simulink library "vmc"  (R2021b)
settings: Solver=VariableStepAuto  StartTime=0.0  StopTime=10.0  RelTol=1e-3
undefined symbols (not defined in the file or in its folder): AVMC_ACCDeltaTqIGain_X_kph, AVMC_ACCDeltaTqIGain_Y_mps2, AVMC_ACCDeltaTqPGain_X_kph, AVMC_ACCDeltaTqPGain_Y_kph, AVMC_ACCLongSteadyCtrl_X_kph, AVMC_AggressJerkPCT4AT_X_kph, AVMC_AggressJerkPCT_X_kph, AVMC_AggressLimitPCT4AT_X_kph, AVMC_AggressLimitPCT_X_kph, AVMC_CCLongSteadyCtrl_X_kph, AVMC_DISCDeltaTqIGain_X_kph, AVMC_DISCDeltaTqIGain_Y_mps2, AVMC_DISCDeltaTqPGain_X_kph, AVMC_DISCDeltaTqPGain_Y_kph, AVMC_DISCTrunAccJerk_X_s, AVMC_DISCTrunAccLimit_X_s, AVMC_ESCRegenOut_X_kph, AVMC_ESCRegenOut_Y_Deg, AVMC_ESCRegenOutEnSpd_X_Deg, AVMC_ISOAccLimit_X_mps, AVMC_ISODecLimit_X_mps, AVMC_ISOJerk_X_mps, AVMC_LatESCRegenOut_X_kph, AVMC_LatESCRegenOut_Y_Deg, AVMC_LongAccDeadZone_X_kph, AVMC_LongAccFiltTsforP2_X_Gps, AVMC_MCPresBaseTq_X_bar, AVMC_MSALongSteadyCtrl_X_kph, AVMC_MSAPedalOvrd2_X_kph, AVMC_MSAPedalOvrd_X_kph, AVMC_MSASpdBand_X_kph, AVMC_MSATqDownEndTq_X_kph, AVMC_MSATqDownTime_X_kph, AVMC_OPDDisSlideRate_X_Deg, AVMC_RDCDetectTime_X_kph, AVMC_RDCDetectTime_Y_pct, AVMC_RDCEnSlideRate_X_Deg, AVMC_RearWhlTqRatio_X_Nm, AVMC_RearWhlTqRatio_Y_gps, AVMC_RearWhlTqSlipGain_X_rat, AVMC_RearWhlTqSlipGain_Y_kph, AVMC_RearWhlTqSTRGGain_X_deg, AVMC_RearWhlTqSTRGGain_Y_kph, AVMC_RWSRrTSA2RWSPos_X_deg, AVMC_RWSSAS2FrtTSA_X_deg, AVMC_RWSVehSPD2RWSCoef_X_kph, AVMC_SoftJerkPCT_X_kph, AVMC_SoftLimitPCT_X_kph, AVMC_StESCYaw_X_kph, AVMC_StESCYaw_Y_Deg, AVMC_StESCYawCom_X_kph, AVMC_StESCYawCom_Y_Gps, AVMC_TMSpdBaseTq_X_rpm, AVMC_VehHoldBDecMap_X_kph, AVMC_VehHoldDecCtrlTime_X_kph, AVMC_VehHoldMCPPass_X_deg, C_TASK_10MS_S, C_TASK_5MS_S, DEG2RAD, ENUM_ACCAVAIL_AVAILABLE ... (+409)
libraries: hcu_lib x74, simulink x68, simulink_extras x3, $bdroot x2
(part 9 of 15)

== system vmc/VMC/VMC/MSA function/MSATorqueSourceDetermination ==
  VVMC_MSAWhlTqCal_Nm : Inport
  VTQD_DriverWhlTqDem_Nm : Inport  Port=2
  VTQD_LowIdleAccPedal_flg : Inport  Port=3
  VDHP_ActAPSPosn_pct : Inport  Port=4
  VINP_VehSpeed_kph : Inport  Port=5
  task_time_s : Inport  Port=6
  VVMC_FeatSetSpdForCalcu_kph : Inport  Port=7
  VVMC_MeterIndSpeedForCalcu_kph : Inport  Port=8
  VVMC_MSAActive_flg : Inport  Port=9
  VTQD_SWCResUpSta_flg : Inport  Port=10
  VVMC_AntiSpdLimEn_flg : Inport  Port=11
  1-D Lookup Table : Lookup_n-D  NumberOfTableDimensions=1  BreakpointsForDimension1=AVMC_MSASpdBand_X_kph  Table=MVMC_MSASpdBand_Y_pct  InternalRulePriority=Speed  RndMeth=Simplest  InputSameDT=on
  1-D Lookup Table1 : Lookup_n-D  NumberOfTableDimensions=1  BreakpointsForDimension1=AVMC_MSASpdBand_X_kph  Table=MVMC_MSASpdBand_Y_pct  InternalRulePriority=Speed  RndMeth=Simplest  InputSameDT=on
  AND : Logic  Inputs=3  AllPortsSameDT=off  OutDataTypeStr=boolean
  AND1 : Logic  AllPortsSameDT=off  OutDataTypeStr=boolean
  AND2 : Logic  AllPortsSameDT=off  OutDataTypeStr=boolean
  Add : Sum  Inputs=+-
  Add1 : Sum  Inputs=+-
  Add11 : Sum  Inputs=+-
  Add2 : Sum
  Cast To Single5 : DataTypeConversion  OutDataTypeStr=single
  Constant : Constant  Value=KVMC_MSAOvrdJudgeSpd_kph
  Constant{1..2,10,16} (4 alike) : Constant  Value=TRUE
  Constant{5,11,17,39} (4 alike) : Constant  Value=FALSE
  Constant12 : Constant  Value=KVMC_MSAWhlTqReqJudgeSW_flg
  Constant13 : Constant  Value=KVMC_MSAOvrdTqRampSlope_Nmps
  Constant14 : Constant  Value=KVMC_MSATqLowLim_Nm  OutDataTypeStr=single
  Constant15 : Constant  Value=KVMC_MSAOvrdTqRampLim_flg  OutDataTypeStr=single
  Constant3 : Constant  Value=KVMC_MSAOvrdDetTime_s
  Constant4 : Constant  Value=KVMC_MSAOvrdResumeTime_s
  Constant{7,9,43,45} (4 alike) : Constant  Value=pct
  Constant49 : Constant  Value=KVMC_MSATqUpLim_Nm  OutDataTypeStr=single
  Constant6 : Constant  Value=KVMC_MSALowIdleAccPedalResOvrd_flg
  Constant8 : Constant  Value=KVMC_MSAOvrdSW_flg
  Detect Decrease : simulink/Logic and Bit Operations/Detect Decrease  vinit=0.0  OutDataTypeStr=boolean
  Detect Increase{,1..3} (4 alike) : simulink/Logic and Bit Operations/Detect Increase  vinit=0.0  OutDataTypeStr=boolean
  Divide : Product  Inputs=**
  Logical Operator : Logic  Inputs=3  AllPortsSameDT=off  OutDataTypeStr=boolean
  Logical Operator1 : Logic  Inputs=5  AllPortsSameDT=off  OutDataTypeStr=boolean
  Logical Operator2 : Logic  Operator=OR  Inputs=3  AllPortsSameDT=off  OutDataTypeStr=boolean
  Logical Operator3 : Logic  Operator=OR  Inputs=4  AllPortsSameDT=off  OutDataTypeStr=boolean
  Logical Operator4 : Logic  AllPortsSameDT=off  OutDataTypeStr=boolean
  Logical Operator5 : Logic  Operator=OR  AllPortsSameDT=off  OutDataTypeStr=boolean
  MVMC_MSAPedalOvrd2_Y_Nm : Lookup_n-D  NumberOfTableDimensions=1  BreakpointsForDimension1=AVMC_MSAPedalOvrd2_X_kph  Table=MVMC_MSAPedalOvrd2_Y_Nm  ExtrapMethod=Clip  InternalRulePriority=Speed  RndMeth=Simplest  InputSameDT=on
  MVMC_MSAPedalOvrd_Y_pct : Lookup_n-D  NumberOfTableDimensions=1  BreakpointsForDimension1=AVMC_MSAPedalOvrd_X_kph  Table=MVMC_MSAPedalOvrd_Y_pct  ExtrapMethod=Clip  InternalRulePriority=Speed  RndMeth=Simplest  InputSameDT=on
  Merge : Merge
  Merge1 : Merge
  Min : MinMax  Inputs=2
  NOT{,1..6} (7 alike) : Logic  Operator=NOT  AllPortsSameDT=off  OutDataTypeStr=boolean
  Product1 : Product
  Product2 : Product  Inputs=*/
  Product6 : Product
  Product7 : Product  Inputs=*/
  Relational Operator{,3,5..6} (4 alike) : RelationalOperator  OutDataTypeStr=boolean  RndMeth=Simplest
  Relational Operator1 : RelationalOperator  Operator=<=  OutDataTypeStr=boolean  RndMeth=Simplest
  Relational Operator2 : RelationalOperator  Operator=>  OutDataTypeStr=boolean  RndMeth=Simplest
  Relational Operator4 : RelationalOperator  Operator=<=  OutDataTypeStr=boolean  RndMeth=Simplest
  Relational Operator7 : RelationalOperator  Operator=<  OutDataTypeStr=boolean  RndMeth=Simplest
  Relational Operator8 : RelationalOperator  Operator=>  OutDataTypeStr=boolean  RndMeth=Simplest
  Saturation Dynamic7 : simulink/Discontinuities/Saturation Dynamic  OutMin=[]  OutMax=[]  OutDataTypeStr=Inherit: Same as second input  OutDataType=fixdt(1, 16)  OutScaling=2^-10  DoSatur=off
  Switch : Switch  Criteria=u2 ~= 0
  Switch{1..6} (6 alike) : Switch  Criteria=u2 > Threshold
  Timer : hcu_lib/Basic_Blocks/Timer
  Timer1 : hcu_lib/Basic_Blocks/Timer
  Triggered Subsystem : Subsystem  TreatAsAtomicUnit=on
  Triggered Subsystem1 : Subsystem  TreatAsAtomicUnit=on
  Triggered Subsystem2 : Subsystem  TreatAsAtomicUnit=on
  Triggered Subsystem3 : Subsystem  TreatAsAtomicUnit=on
  Unit Delay{,1..3} (4 alike) : UnitDelay  SampleTime=-1  HasFrameUpgradeWarning=on
  VVMC_MSAWhlTqReq_Nm : Outport
  VVMC_MSAOvrdAllow_flg : Outport  Port=2
  VVMC_MSAWhlTqActive_flg : Outport  Port=3
  wires:
  Switch3/1 -> Switch1/2, Switch/2
  [VVMC_MSAWhlTqActive_flg] -> VVMC_MSAWhlTqActive_flg/1
  Switch1/1 -> [VVMC_MSAWhlTqActive_flg]  "VVMC_MSAWhlTqActive_flg"
  Constant10/1 -> Switch1/3
  Constant11/1 -> Switch1/1
  Relational Operator7/1 -> AND1/2
  Add1/1 -> Product2/1
  Constant7/1 -> Add1/1
  Constant9/1 -> Product2/2
  1-D Lookup Table1/1 -> Add1/2
  [VVMC_FeatSetSpdForCalcu_kph] -> Product1/1
  Product1/1 -> Relational Operator7/2
  [VVMC_MeterIndSpeedForCalcu_kph] -> Relational Operator7/1
  Product2/1 -> Product1/2
  Relational Operator6/1 -> Logical Operator1/5
  Product6/1 -> Relational Operator6/2
  [VVMC_FeatSetSpdForCalcu_kph] -> Product6/1
  Constant45/1 -> Product7/2
  Product7/1 -> Product6/2
  [VVMC_MeterIndSpeedForCalcu_kph] -> Relational Operator6/1
  1-D Lookup Table/1 -> Add11/2
  Add11/1 -> Product7/1
  Constant43/1 -> Add11/1
  [VVMC_MSAActive_flg] -> NOT5/1
  NOT5/1 -> Logical Operator3/2
  [VVMC_MSAActive_flg] -> Logical Operator1/1
  NOT4/1 -> Logical Operator5/2
  Logical Operator5/1 -> Triggered Subsystem1/Trigger
  [VVMC_MSAActive_flg] -> NOT4/1
  [VVMC_MSAActive_flg] -> Logical Operator/1
  VVMC_MSAActive_flg/1 -> [VVMC_MSAActive_flg]
  Constant6/1 -> Logical Operator4/2
  Logical Operator4/1 -> Logical Operator3/3
  Triggered Subsystem2/2(Out2) -> Merge1/1
  Triggered Subsystem3/1(Out1) -> Merge1/2
  Constant5/1 -> Triggered Subsystem3/1(In1)
  Detect Increase2/1 -> Triggered Subsystem3/Trigger
  Relational Operator5/1 -> Detect Increase2/1
  Timer1/1 -> Relational Operator5/1
  Constant4/1 -> Timer1/4, Relational Operator5/2
  [task_time_s] -> Timer1/3
  NOT3/1 -> Timer1/2
  [VVMC_MSAOvrdProhibit_flg] -> Logical Operator3/4
  [VTQD_LowIdleAccPedal_flg] -> Logical Operator4/1
  Logical Operator3/1 -> Timer1/1, NOT3/1
  Relational Operator4/1 -> Logical Operator3/1
  VVMC_MeterIndSpeedForCalcu_kph/1 -> [VVMC_MeterIndSpeedForCalcu_kph]
  [VVMC_MeterIndSpeedForCalcu_kph] -> Relational Operator4/1
  [VVMC_FeatSetSpdForCalcu_kph] -> Relational Operator4/2
  Constant1/1 -> Triggered Subsystem2/2(In2)
  Detect Increase1/1 -> Triggered Subsystem2/Trigger
  Relational Operator3/1 -> Detect Increase1/1
  [VVMC_MSAOvrdAllow_flg] -> VVMC_MSAOvrdAllow_flg/1
  Timer/1 -> Relational Operator3/1
  VVMC_FeatSetSpdForCalcu_kph/1 -> [VVMC_FeatSetSpdForCalcu_kph]
  MVMC_MSAPedalOvrd_Y_pct/1 -> Relational Operator2/2  "VVMC_MSAPedalOvrd_pct"
  [VVMC_FeatSetSpdForCalcu_kph] -> MVMC_MSAPedalOvrd_Y_pct/1
  [VVMC_MSAOvrdAllow_flg] -> Logical Operator2/1
  Merge1/1 -> [VVMC_MSAOvrdAllow_flg]  "VVMC_MSAOvrdAllow_flg"
  Constant3/1 -> Timer/4, Relational Operator3/2
  [task_time_s] -> Timer/3
  task_time_s/1 -> [task_time_s]
  NOT2/1 -> Timer/2
  NOT1/1 -> Logical Operator1/3
  [VVMC_MSAOvrdProhibit_flg] -> NOT1/1
  Logical Operator1/1 -> Timer/1, NOT2/1
  [VTQD_LowIdleAccPedal_flg] -> NOT/1
  NOT/1 -> Logical Operator1/2
  Relational Operator2/1 -> Switch2/3
  [VDHP_ActAPSPosn_pct] -> Relational Operator2/1
  Switch6/1 -> [VVMC_MSAOvrdProhibit_flg]  "VVMC_MSAOvrdProhibit_flg"
  Triggered Subsystem/1(Out1) -> Merge/1
  Triggered Subsystem1/1(Out1) -> Merge/2
  Constant39/1 -> Triggered Subsystem1/1(In1)
  Detect Increase/1 -> Logical Operator5/1
  [VTQD_LowIdleAccPedal_flg] -> Detect Increase/1
  Constant2/1 -> Triggered Subsystem/1(In1)
  Logical Operator/1 -> Triggered Subsystem/Trigger
  Detect Decrease/1 -> Logical Operator/2
  Relational Operator1/1 -> Logical Operator/3
  Constant/1 -> Relational Operator1/2
  [VINP_VehSpeed_kph] -> Relational Operator1/1
  [VTQD_LowIdleAccPedal_flg] -> Detect Decrease/1
  VINP_VehSpeed_kph/1 -> [VINP_VehSpeed_kph]
  VDHP_ActAPSPosn_pct/1 -> [VDHP_ActAPSPosn_pct]
  VTQD_LowIdleAccPedal_flg/1 -> [VTQD_LowIdleAccPedal_flg]
  VTQD_DriverWhlTqDem_Nm/1 -> [VTQD_DriverWhlTqDem_Nm]
  VVMC_MSAWhlTqCal_Nm/1 -> [VVMC_MSAWhlTqCal_Nm]
  [VVMC_MSAWhlTqReq_Nm] -> VVMC_MSAWhlTqReq_Nm/1
  Switch/1 -> [VVMC_MSAWhlTqReq_Nm], Unit Delay1/1  "VVMC_MSAWhlTqReq_Nm"
  [VVMC_MSAWhlTqCal_Nm] -> Switch/3
  [VTQD_DriverWhlTqDem_Nm] -> Relational Operator/2
  Relational Operator/1 -> Logical Operator2/3
  [VVMC_MSAWhlTqCal_Nm] -> Relational Operator/1
  [VTQD_DriverWhlTqDem_Nm] -> Switch4/3
  AND1/1 -> Logical Operator2/2
  VTQD_SWCResUpSta_flg/1 -> [VTQD_SWCResUpSta_flg]
  [VVMC_MSAWhlTqActive_flg] -> Unit Delay/1
  Unit Delay/1 -> AND/1
  [VTQD_SWCResUpSta_flg] -> AND/2
  AND/1 -> Switch3/2
  Constant17/1 -> Switch3/1
  Logical Operator2/1 -> Switch3/3
  [VVMC_FeatSetSpdForCalcu_kph] -> 1-D Lookup Table/1
  [VVMC_FeatSetSpdForCalcu_kph] -> 1-D Lookup Table1/1
  NOT6/1 -> AND/3
  [VTQD_LowIdleAccPedal_flg] -> NOT6/1
  Constant12/1 -> AND1/1
  Switch2/1 -> Logical Operator1/4
  Constant8/1 -> Switch2/2
  [VVMC_FeatSetSpdForCalcu_kph] -> MVMC_MSAPedalOvrd2_Y_Nm/1
  MVMC_MSAPedalOvrd2_Y_Nm/1 -> Relational Operator8/2
  Relational Operator8/1 -> Switch2/1
  [VTQD_DriverWhlTqDem_Nm] -> Add/1
  Add/1 -> Relational Operator8/1
  [VVMC_MSAWhlTqCal_Nm] -> Unit Delay3/1
  Unit Delay1/1 -> [VVMC_LastMSAWhlTqReq_Nm]
  [VVMC_MSAOvrdAllow_flg] -> AND2/1
  Switch4/1 -> Switch/1
  [VVMC_MSAOvrdEnTq_Nm] -> Switch5/1
  Constant13/1 -> Divide/1
  [task_time_s] -> Divide/2
  Divide/1 -> Add2/2
  Constant14/1 -> Saturation Dynamic7/3
  Add2/1 -> Cast To Single5/1
  Constant49/1 -> Saturation Dynamic7/1
  Cast To Single5/1 -> Saturation Dynamic7/2
  Saturation Dynamic7/1 -> Unit Delay2/1, Min/1
  [VTQD_DriverWhlTqDem_Nm] -> Min/2
  Min/1 -> Switch4/1
  [VVMC_LastMSAWhlTqReq_Nm] -> Triggered Subsystem2/1(In1)
  Triggered Subsystem2/1(Out1) -> [VVMC_MSAOvrdEnTq_Nm]
  [VVMC_MSAOvrdAllow_flg] -> Detect Increase3/1
  Detect Increase3/1 -> Switch5/2
  Switch5/1 -> Add2/1
  Unit Delay2/1 -> Switch5/3
  Constant15/1 -> AND2/2
  AND2/1 -> Switch4/2
  Unit Delay3/1 -> Add/2
  VVMC_AntiSpdLimEn_flg/1 -> [VVMC_AntiSpdLimEn_flg]
  [VVMC_AntiSpdLimEn_flg] -> Switch6/2
  Merge/1 -> Switch6/3
  Constant16/1 -> Switch6/1

== system vmc/VMC/VMC/RDC Determination/RWD ==
  task_time_s : Inport
  VVMC_ActMaxSlideRate_pct : Inport  Port=2
  VTQD_AfterAvailableTqDemFr_Nm : Inport  Port=3
  VTQD_AfterAvailableTqDemRr_Nm : Inport  Port=4
  VINP_ESCActive_flg : Inport  Port=5
  VINP_SASAngle_Deg : Inport  Port=6
  VINP_LatAccel_Gps : Inport  Port=7
  VINP_VehSpeed_kph : Inport  Port=8
  VINP_YawRate_degps : Inport  Port=9
  VINP_RDCActive_enum : Inport  Port=10
  VINP_DIDGetDynoMode_flg : Inport  Port=11
  AND{,2..5} (5 alike) : Logic  AllPortsSameDT=off  OutDataTypeStr=boolean
  AND1 : Logic  Inputs=3  AllPortsSameDT=off  OutDataTypeStr=boolean
  Abs{,1..7} (8 alike) : Abs
  Add1 : Sum
  Constant1 : Constant  Value=ZERO_INT
  Constant2 : Constant  Value=KVMC_DIDGetDynoModeSW_flg
  Constant{3..4,74,78} (4 alike) : Constant  Value=KVMC_AltRDCActiveTq_Nm
  Constant73 : Constant  Value=ENUM_RDCACTSTA_NOREQUEST
  Constant77 : Constant  Value=ENUM_RDCACTSTA_RAMPOUT
  Constant81 : Constant  Value=KVMC_AltRDCActiveSW_flg
  Constant82 : Constant  Value=ENUM_RDCACTSTA_EXITIMMEDIATELY
  Constant83 : Constant  Value=KVMC_AltRDCRecTime_s
  Constant86 : Constant  Value=KVMC_ESCRegenTqRecDelay_s
  Constant95 : Constant  Value=ENUM_RDCACTSTA_EXITIMMEDIATELY
  Delay{1..2,6..7} (4 alike) : Delay  DelayLength=1
  DelayEnable1 : hcu_lib/Basic_Blocks/DelayEnable
  DelayEnable2 : hcu_lib/Basic_Blocks/DelayEnable
  DelayEnable3 : hcu_lib/Basic_Blocks/DelayEnable
  Equal33 : RelationalOperator  Operator===  OutDataTypeStr=boolean  RndMeth=Simplest
  MVMC_ESCRegenOutEnSpd_Y_kph : Lookup_n-D  NumberOfTableDimensions=1  BreakpointsForDimension1=AVMC_ESCRegenOutEnSpd_X_Deg  Table=MVMC_ESCRegenOutEnSpd_Y_kph  ExtrapMethod=Clip  InternalRulePriority=Speed  RndMeth=Simplest  InputSameDT=on
  MVMC_ESCRegenOut_Z_Dps : Lookup_n-D  BreakpointsForDimension1=AVMC_ESCRegenOut_Y_Deg  BreakpointsForDimension2=AVMC_ESCRegenOut_X_kph  Table=MVMC_ESCRegenOut_Z_Dps  ExtrapMethod=Clip  InternalRulePriority=Speed  RndMeth=Simplest  InputSameDT=on
      settings: InputPortMap=u0,u1
  MVMC_LatESCRegenOut_Z_Gps : Lookup_n-D  BreakpointsForDimension1=AVMC_LatESCRegenOut_Y_Deg  BreakpointsForDimension2=AVMC_LatESCRegenOut_X_kph  Table=MVMC_LatESCRegenOut_Z_Gps  ExtrapMethod=Clip  InternalRulePriority=Speed  RndMeth=Simplest  InputSameDT=on
      settings: InputPortMap=u0,u1
  MVMC_RDCDetectTime_Z_s : Lookup_n-D  BreakpointsForDimension1=AVMC_RDCDetectTime_Y_pct  BreakpointsForDimension2=AVMC_RDCDetectTime_X_kph  Table=MVMC_RDCDetectTime_Z_s  ExtrapMethod=Clip  InternalRulePriority=Speed  RndMeth=Simplest  InputSameDT=on
      settings: InputPortMap=u0,u1
  MVMC_RDCEnSlideRate_Y_pct : Lookup_n-D  NumberOfTableDimensions=1  BreakpointsForDimension1=AVMC_RDCEnSlideRate_X_Deg  Table=MVMC_RDCEnSlideRate_Y_pct  ExtrapMethod=Clip  InternalRulePriority=Speed  RndMeth=Simplest  InputSameDT=on
  MVMC_StESCYawCom_Z_Dps : Lookup_n-D  BreakpointsForDimension1=AVMC_StESCYawCom_Y_Gps  BreakpointsForDimension2=AVMC_StESCYawCom_X_kph  Table=MVMC_StESCYawCom_Z_Dps  ExtrapMethod=Clip  InternalRulePriority=Speed  RndMeth=Simplest  InputSameDT=on
      settings: InputPortMap=u0,u1
  MVMC_StESCYaw_Z_Dps : Lookup_n-D  BreakpointsForDimension1=AVMC_StESCYaw_Y_Deg  BreakpointsForDimension2=AVMC_StESCYaw_X_kph  Table=MVMC_StESCYaw_Z_Dps  ExtrapMethod=Clip  InternalRulePriority=Speed  RndMeth=Simplest  InputSameDT=on
      settings: InputPortMap=u0,u1
  NOT : Logic  Operator=NOT  AllPortsSameDT=off  OutDataTypeStr=boolean
  NOT1 : Logic  Operator=NOT  AllPortsSameDT=off  OutDataTypeStr=boolean
  NOT3 : Logic  Operator=NOT  AllPortsSameDT=off  OutDataTypeStr=boolean
  OR{,1..4,9} (6 alike) : Logic  Operator=OR  AllPortsSameDT=off  OutDataTypeStr=boolean
  OR8 : Logic  AllPortsSameDT=off  OutDataTypeStr=boolean
  Relational Operator{1,8..10} (4 alike) : RelationalOperator  OutDataTypeStr=boolean  RndMeth=Simplest
  Relational Operator{2..7} (6 alike) : RelationalOperator  Operator=<=  OutDataTypeStr=boolean  RndMeth=Simplest
  SR_Latch4 : hcu_lib/Basic_Blocks/SR_Latch
  SR_Latch5 : hcu_lib/Basic_Blocks/SR_Latch
  Switch10 : Switch  Criteria=u2 > Threshold
  Switch11 : Switch  Criteria=u2 > Threshold
  Switch8 : Switch  Criteria=u2 > Threshold
  VVMC_RWDRDCActive_enum : Outport
  VVMC_RDCEnSlideRate_pct : Outport  Port=2
  VVMC_ActStESCYaw_Dps : Outport  Port=3
  wires:
  [VVMC_RDCDetectTime_s] -> DelayEnable1/2
  MVMC_RDCEnSlideRate_Y_pct/1 -> VVMC_RDCEnSlideRate_pct/1, [VVMC_RDCEnSlideRate_pct]  "VVMC_RDCEnSlideRate_pct"
  VINP_YawRate_degps/1 -> [VINP_YawRate_degps]
  [VINP_ESCActive_flg] -> NOT1/1
  VINP_ESCActive_flg/1 -> [VINP_ESCActive_flg]
  OR2/1 -> AND3/1
  Constant73/1 -> Switch8/3
  Delay7/1 -> Relational Operator3/1
  VINP_LatAccel_Gps/1 -> [VINP_LatAccel_Gps]
  [VVMC_RDCEnSlideRate_pct] -> Relational Operator1/2
  Switch11/1 -> [VVMC_AltRDCActive_enum]  "VVMC_AltRDCActive_enum"
  VINP_VehSpeed_kph/1 -> [VINP_VehSpeed_kph]
  Constant78/1 -> Relational Operator3/2
  [VINP_SASAngle_Deg] -> Abs7/1
  VVMC_ActMaxSlideRate_pct/1 -> [VVMC_ActMaxSlideRate_pct]
  DelayEnable2/1 -> OR3/2  "VVMC_AltRDCRec_flg"
  [task_time_s] -> DelayEnable1/3
  OR9/1 -> AND4/1
  [VINP_SASAngle_Deg] -> MVMC_LatESCRegenOut_Z_Gps/1
  [VVMC_ActMaxSlideRate_pct] -> MVMC_RDCDetectTime_Z_s/1
  [VINP_LatAccel_Gps] -> Abs5/1
  VTQD_AfterAvailableTqDemRr_Nm/1 -> [VTQD_AfterAvailableTqDemRr_Nm]
  SR_Latch5/1 -> [VVMC_ESCActive_flg]  "VVMC_ESCActive_flg"
  Abs4/1 -> Relational Operator8/1
  DelayEnable1/1 -> SR_Latch4/1  "VVMC_RDCDetectEn_flg"
  Relational Operator8/1 -> OR9/2
  Constant74/1 -> Relational Operator2/2
  [VVMC_ESCSlip_flg] -> SR_Latch5/1
  Abs5/1 -> Relational Operator10/1
  [VINP_SASAngle_Deg] -> MVMC_ESCRegenOut_Z_Dps/1
  [VINP_VehSpeed_kph] -> Relational Operator9/1
  Switch8/1 -> Switch11/3
  NOT3/1 -> OR8/1
  [VTQD_AfterAvailableTqDemFr_Nm] -> Delay6/1
  Delay6/1 -> Relational Operator2/1
  MVMC_RDCDetectTime_Z_s/1 -> [VVMC_RDCDetectTime_s]  "VVMC_RDCDetectTime_s"
  [VTQD_AfterAvailableTqDemRr_Nm] -> Delay7/1
  [VINP_SASAngle_Deg] -> MVMC_RDCEnSlideRate_Y_pct/1
  AND3/1 -> DelayEnable1/1
  [VVMC_ESCActive_flg] -> OR4/1
  Relational Operator3/1 -> OR2/2
  Relational Operator9/1 -> AND4/2, AND1/1
  Relational Operator1/1 -> AND3/2
  MVMC_ESCRegenOut_Z_Dps/1 -> Relational Operator8/2  "VVMC_ESCRegenOut_Dps"
  [VINP_YawRate_degps] -> Abs4/1
  SR_Latch4/1 -> Switch8/2
  [VVMC_ActMaxSlideRate_pct] -> Abs2/1
  Switch10/1 -> VVMC_RWDRDCActive_enum/1  "VVMC_RWDRDCActive_enum"
  [VINP_RDCActive_enum] -> Equal33/1
  VINP_SASAngle_Deg/1 -> [VINP_SASAngle_Deg]
  [task_time_s] -> DelayEnable3/3
  Abs2/1 -> Relational Operator1/1
  MVMC_LatESCRegenOut_Z_Gps/1 -> Relational Operator10/2  "VVMC_LatESCRegenOut_Gps"
  NOT1/1 -> OR8/2
  Equal33/1 -> OR4/2
  [VINP_VehSpeed_kph] -> MVMC_LatESCRegenOut_Z_Gps/2
  [VVMC_ESCSlip_flg] -> NOT3/1
  Relational Operator2/1 -> OR2/1
  Relational Operator10/1 -> OR9/1
  Constant95/1 -> Switch11/1
  [VINP_VehSpeed_kph] -> MVMC_ESCRegenOut_Z_Dps/2
  OR8/1 -> DelayEnable3/1
  OR4/1 -> Switch11/2
  [VVMC_AltRDCActive_enum] -> Switch10/1
  DelayEnable3/1 -> SR_Latch5/2
  Constant77/1 -> Switch8/1
  Constant86/1 -> DelayEnable3/2
  Constant82/1 -> Equal33/2
  VTQD_AfterAvailableTqDemFr_Nm/1 -> [VTQD_AfterAvailableTqDemFr_Nm]
  VINP_RDCActive_enum/1 -> [VINP_RDCActive_enum]
  task_time_s/1 -> [task_time_s]
  Constant1/1 -> Switch10/3
  [VINP_LatAccel_Gps] -> Abs1/1
  [VINP_SASAngle_Deg] -> Abs/1
  Abs/1 -> MVMC_StESCYaw_Z_Dps/1
  Add1/1 -> VVMC_ActStESCYaw_Dps/1, [VVMC_ActStESCYaw_Dps]  "VVMC_ActStESCYaw_Dps"
  MVMC_StESCYaw_Z_Dps/1 -> Add1/1  "VVMC_StESCYaw_Dps"
  [VINP_VehSpeed_kph] -> MVMC_StESCYaw_Z_Dps/2
  [VINP_VehSpeed_kph] -> MVMC_StESCYawCom_Z_Dps/2
  MVMC_StESCYawCom_Z_Dps/1 -> Add1/2  "VVMC_StESCYawCom_Dps"
  Abs1/1 -> MVMC_StESCYawCom_Z_Dps/1
  [VINP_VehSpeed_kph] -> MVMC_RDCDetectTime_Z_s/2
  AND/1 -> DelayEnable2/1
  [task_time_s] -> DelayEnable2/3
  Relational Operator4/1 -> AND/1
  [VVMC_ActStESCYaw_Dps] -> Relational Operator6/2
  [VVMC_RDCEnSlideRate_pct] -> Relational Operator4/2
  Abs6/1 -> Relational Operator6/1
  Relational Operator6/1 -> AND/2
  Abs3/1 -> Relational Operator4/1
  [VVMC_ActMaxSlideRate_pct] -> Abs3/1
  Constant83/1 -> DelayEnable2/2
  [VINP_YawRate_degps] -> Abs6/1
  Abs7/1 -> MVMC_ESCRegenOutEnSpd_Y_kph/1
  MVMC_ESCRegenOutEnSpd_Y_kph/1 -> Relational Operator9/2  "VVMC_ESCRegenOutEnSpd_kph"
  Constant4/1 -> Relational Operator7/2
  Delay1/1 -> Relational Operator5/1
  [VTQD_AfterAvailableTqDemRr_Nm] -> Delay2/1
  Constant3/1 -> Relational Operator5/2
  Delay2/1 -> Relational Operator7/1
  Relational Operator7/1 -> OR1/2
  Relational Operator5/1 -> OR1/1
  [VTQD_AfterAvailableTqDemFr_Nm] -> Delay1/1
  OR1/1 -> AND1/3
  [VINP_ESCActive_flg] -> AND1/2
  AND4/1 -> OR/1
  AND1/1 -> OR/2
  OR/1 -> [VVMC_ESCSlip_flg]  "VVMC_ESCSlip_flg"
  Constant81/1 -> AND2/1
  AND2/1 -> Switch10/2
  VINP_DIDGetDynoMode_flg/1 -> [VINP_DIDGetDynoMode_flg]
  [VINP_DIDGetDynoMode_flg] -> AND5/1
  Constant2/1 -> AND5/2
  AND5/1 -> NOT/1
  NOT/1 -> AND2/2
  [VINP_ESCActive_flg] -> OR3/1
  OR3/1 -> SR_Latch4/2

== system vmc/VMC/VMC/SPD2ACC/ISO22179 ==
  VVMC_MeterSpdCalcu_mps : Inport
  VVMC_LimitPCT_pct : Inport  Port=2
  Constant : Constant  Value=pct
  Constant1 : Constant  Value=MINUSONE_FLOAT
  Divide : Product  Inputs=**
  Divide1 : Product  Inputs=**
  Divide2 : Product  Inputs=*/
  Divide3 : Product  Inputs=**
  MVMC_ISOAccLimit_Y_mps2 : Lookup_n-D  NumberOfTableDimensions=1  BreakpointsForDimension1=AVMC_ISOAccLimit_X_mps  UseOneInputPortForAllInputData=on  Table=MVMC_ISOAccLimit_Y_mps2  UseLastTableValue=on  InternalRulePriority=Speed  RndMeth=Simplest  InputSameDT=on
  MVMC_ISODecLimit_Y_mps2 : Lookup_n-D  NumberOfTableDimensions=1  BreakpointsForDimension1=AVMC_ISODecLimit_X_mps  UseOneInputPortForAllInputData=on  Table=MVMC_ISODecLimit_Y_mps2  UseLastTableValue=on  InternalRulePriority=Speed  RndMeth=Simplest  InputSameDT=on
  MVMC_ISOJerk_Y_mps3 : Lookup_n-D  NumberOfTableDimensions=1  BreakpointsForDimension1=AVMC_ISOJerk_X_mps  UseOneInputPortForAllInputData=on  Table=MVMC_ISOJerk_Y_mps3  UseLastTableValue=on  InternalRulePriority=Speed  RndMeth=Simplest  InputSameDT=on
  VVMC_ISOAccLimit_mps2 : Outport
  VVMC_ISODecLimit_mps2 : Outport  Port=2
  VVMC_ISOJerkLimit_mps3 : Outport  Port=3
  wires:
  Constant1/1 -> Divide3/1
  [VVMC_ISOJerkLimit_mps3] -> VVMC_ISOJerkLimit_mps3/1  "VVMC_ISOJerkLimit_mps3"
  [VVMC_ISODecLimit_mps2] -> VVMC_ISODecLimit_mps2/1  "VVMC_ISODecLimit_mps2"
  [VVMC_ISOAccLimit_mps2] -> VVMC_ISOAccLimit_mps2/1  "VVMC_ISOAccLimit_mps2"
  [VVMC_MeterSpdCalcu_mps] -> MVMC_ISOJerk_Y_mps3/1
  Constant/1 -> Divide2/2
  [VVMC_LimitPCT_pct] -> Divide2/1
  VVMC_LimitPCT_pct/1 -> [VVMC_LimitPCT_pct]
  VVMC_MeterSpdCalcu_mps/1 -> [VVMC_MeterSpdCalcu_mps]
  Divide/1 -> [VVMC_ISOAccLimit_mps2]
  MVMC_ISOJerk_Y_mps3/1 -> [VVMC_ISOJerkLimit_mps3]
  Divide1/1 -> [VVMC_ISODecLimit_mps2]
  MVMC_ISOAccLimit_Y_mps2/1 -> Divide/2
  [VVMC_MeterSpdCalcu_mps] -> MVMC_ISODecLimit_Y_mps2/1
  Divide3/1 -> Divide1/1
  Divide2/1 -> Divide1/2, Divide/1
  MVMC_ISODecLimit_Y_mps2/1 -> Divide3/2
  [VVMC_MeterSpdCalcu_mps] -> MVMC_ISOAccLimit_Y_mps2/1

== system vmc/VMC/VMC/SPD2ACC/PID ==
  VVMC_SPD2ACCAct_flg : Inport
  VVMC_FeatReqSpd_kph : Inport  Port=2
  VINP_VehSpeed_kph : Inport  Port=3
  VVMC_MeterIndSpeedForCalcu_kph : Inport  Port=4
  Cast To Single : DataTypeConversion  OutDataTypeStr=single
  Constant1 : Constant  Value=ZERO_FLOAT
  Constant10 : Constant  Value=ONE_FLOAT
  Constant2 : Constant  Value=KPH2MPS
  Constant3 : Constant  Value=KPH2MPS
  Constant4 : Constant  Value=ZERO_FLOAT
  Constant5 : Constant  Value=KVMC_PParm_enum
  Constant6 : Constant  Value=KVMC_IParm_enum
  Constant7 : Constant  Value=KVMC_CMDCycleTime_s
  Constant8 : Constant  Value=ZERO_FLOAT
  Constant9 : Constant  Value=KVMC_AccelIGain_enum
  Divide{,1..2,4..5} (5 alike) : Product  Inputs=**
  Divide3 : Product  Inputs=*/
  InitialCondition: 0 : UnitDelay  SampleTime=-1  HasFrameUpgradeWarning=on
  Subtract : Sum
  Sum1 : Sum  Inputs=|+-
  Sum2 : Sum  Inputs=|+-
  Sum4 : Sum  Inputs=|++
  u2 > 0 : Switch  Criteria=u2 > Threshold
  u2 > 0 (1) : Switch  Criteria=u2 > Threshold
  u2 > 0 (2) : Switch  Criteria=u2 > Threshold
  u2 >= 0 : Switch
  VVMC_AccCalcuPID_mps2 : Outport
  VVMC_MeterSpdCalcu_mps : Outport  Port=2
  wires:
  Divide4/1 -> [VVMC_MeterSpdCalcu_mps]
  Constant7/1 -> Cast To Single/1
  Cast To Single/1 -> Divide3/2
  Sum4/1 -> Divide1/2
  Constant8/1 -> u2 > 0 (2)/3
  Constant1/1 -> u2 > 0 (1)/3
  [VVMC_MeterIndSpeedForCalcu_kph] -> Sum1/2, Divide4/1
  Divide3/1 -> [VVMC_AccCalcuPID_mps2]
  Divide/1 -> Subtract/2
  u2 > 0 (1)/1 -> Divide/1
  [VVMC_SPD2ACCAct_flg] -> u2 > 0 (1)/2
  Constant5/1 -> Divide/2
  Divide2/1 -> Divide3/1
  Constant3/1 -> Divide4/2
  [VINP_VehSpeed_kph] -> Sum2/2
  Sum1/1 -> u2 > 0 (2)/2, u2 > 0 (1)/1
  Divide1/1 -> Subtract/1
  Subtract/1 -> Divide2/1
  u2 > 0 (2)/1 -> u2 >= 0/1
  [VVMC_SPD2ACCAct_flg] -> u2 > 0/2
  Constant6/1 -> Divide5/2
  Sum2/1 -> u2 > 0/1, u2 >= 0/2
  [VVMC_FeatReqSpd_kph] -> Sum2/1
  u2 > 0/1 -> Sum4/1, InitialCondition: 0/1
  Constant4/1 -> u2 > 0/3
  InitialCondition: 0/1 -> Sum4/2
  Divide5/1 -> Divide1/1
  Constant2/1 -> Divide2/2
  Constant10/1 -> u2 >= 0/3
  Constant9/1 -> u2 > 0 (2)/1
  u2 >= 0/1 -> Divide5/1
  [VVMC_FeatReqSpd_kph] -> Sum1/1
  VINP_VehSpeed_kph/1 -> [VINP_VehSpeed_kph]
  [VVMC_MeterSpdCalcu_mps] -> VVMC_MeterSpdCalcu_mps/1  "VVMC_MeterSpdCalcu_mps"
  [VVMC_AccCalcuPID_mps2] -> VVMC_AccCalcuPID_mps2/1  "VVMC_AccCalcuPID_mps2"
  VVMC_MeterIndSpeedForCalcu_kph/1 -> [VVMC_MeterIndSpeedForCalcu_kph]
  VVMC_FeatReqSpd_kph/1 -> [VVMC_FeatReqSpd_kph]
  VVMC_SPD2ACCAct_flg/1 -> [VVMC_SPD2ACCAct_flg]
